simulink model "flocking"  (R2018b)
settings: Solver=FixedStepAuto  StartTime=0.0  StopTime=10  FixedStep=continuous_h  RelTol=1e-3
undefined symbols (not defined in the file or in its folder): continuous_h, traj
libraries: simulink x3, cf_lib x1, flocking_lib x1, vel_controller_lib x1
settings Model: Creator=sebbe  LastModifiedBy=sebbe

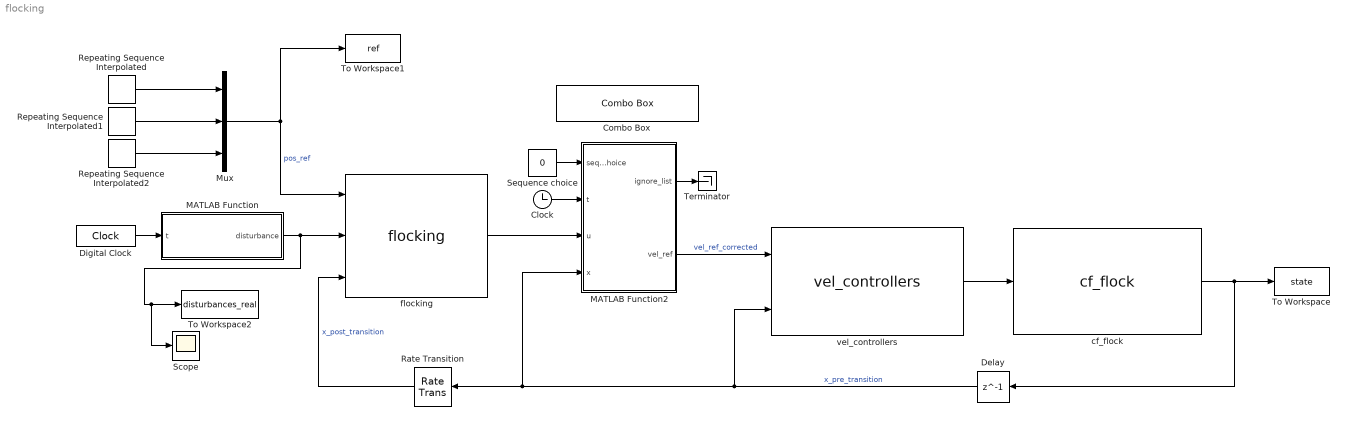
== system flocking ==
  Clock : Clock
  Combo Box : ComboBox  WebBlockId=48  SelectedLabel=Disabled
      settings: Values={{'Disabled', 'Merge 2', 'Fly Through', 'Hover'}, [0 1 2 3]}
  Delay : Delay  DelayLength=1
  Digital Clock : DigitalClock  SampleTime=continuous_h
  MATLAB Function : MATLAB Function  TreatAsAtomicUnit=on
  MATLAB Function2 : MATLAB Function  TreatAsAtomicUnit=on
  Mux : Mux  Inputs=3
  Rate Transition : RateTransition  OutPortSampleTime=0.05
  Repeating Sequence Interpolated : simulink/Sources/Repeating Sequence Interpolated  OutValues=traj.seq(1,:)'  TimeValues=traj.seq_t'  LookUpMeth=Interpolation-Use End Values  tsamp=continuous_h  OutMin=[]  OutMax=[]  OutDataTypeStr=double  OutputDataTypeScalingMode=double  OutDataType=fixdt(0,8)  OutScaling=2^-10
  Repeating Sequence Interpolated1 : simulink/Sources/Repeating Sequence Interpolated  OutValues=traj.seq(2,:)'  TimeValues=traj.seq_t'  LookUpMeth=Interpolation-Use End Values  tsamp=continuous_h  OutMin=[]  OutMax=[]  OutDataTypeStr=double  OutputDataTypeScalingMode=double  OutDataType=fixdt(0,8)  OutScaling=2^-10
  Repeating Sequence Interpolated2 : simulink/Sources/Repeating Sequence Interpolated  OutValues=traj.seq(3,:)'  TimeValues=traj.seq_t'  LookUpMeth=Interpolation-Use End Values  tsamp=continuous_h  OutMin=[]  OutMax=[]  OutDataTypeStr=double  OutputDataTypeScalingMode=double  OutDataType=fixdt(0,8)  OutScaling=2^-10
  Scope : Scope
  Sequence choice : Constant  Value=0
  Terminator : Terminator
  To Workspace : ToWorkspace  VariableName=state  SaveFormat=Timeseries  SampleTime=continuous_h
  To Workspace1 : ToWorkspace  VariableName=ref  SaveFormat=Timeseries  SampleTime=continuous_h
  To Workspace2 : ToWorkspace  VariableName=disturbances_real  SaveFormat=Timeseries  SampleTime=-1
  cf_flock : cf_lib/cf_flock  SystemSampleTime=-1
  flocking : flocking_lib/flocking  SystemSampleTime=-1
  vel_controllers : vel_controller_lib/vel_controllers  SystemSampleTime=-1
  wires:
  vel_controllers/1 -> cf_flock/1
  cf_flock/1 -> Delay/1, To Workspace/1
  Delay/1 -> vel_controllers/2, MATLAB Function2/4(x), Rate Transition/1  "x_pre_transition"
  Repeating Sequence Interpolated1/1 -> Mux/2
  Mux/1 -> flocking/1, To Workspace1/1  "pos_ref"
  Repeating Sequence Interpolated2/1 -> Mux/3
  Repeating Sequence Interpolated/1 -> Mux/1
  Digital Clock/1 -> MATLAB Function/1(t)
  MATLAB Function/1(disturbance) -> flocking/2, Scope/1, To Workspace2/1
  Clock/1 -> MATLAB Function2/2(t)
  MATLAB Function2/2(vel_ref) -> vel_controllers/1  "vel_ref_corrected"
  Sequence choice/1 -> MATLAB Function2/1(sequence_choice)
  Rate Transition/1 -> flocking/3  "x_post_transition"
  flocking/1 -> MATLAB Function2/3(u)
  MATLAB Function2/1(ignore_list) -> Terminator/1

== matlab function flocking/MATLAB Function ==
  data: t input; disturbances parameter; disturbance output
function disturbance = dynamic_disturbance(t, disturbances)
disturbance = disturbances;
%disturbance(3,1) = disturbances(3,1) - 49.6 + 30*t - 9.82*t^2/2;
%disturbance(1,1) = disturbances(1,1) - 3 + 1*t;

== matlab function flocking/MATLAB Function2 ==
  data: ignore_list output; sequence_choice input; t input; u input; vel_ref output; x input
function [ignore_list, vel_ref] = intercept_ref(sequence_choice, t, u, x)
vel_ref = u;
ignore_list = [0];
if sequence_choice == 0
    return
end

[n_states, N] = size(x);

switch sequence_choice
    case 1 % Merge 2
        if t < 6
            r = [0; -1; 1];
            e = r - x(1:3,1);
            vel_ref(:,1) = 0.5*e;
        end
        
    case 2 % Fly through
        r = [2; 0; 1];
        e = r - x(1:3,1);
        vel_ref(:,1) = 0.5*e;
    case 3 % Hover
        pos_hover = [0 0 0.96;
            0.52 0 1.02;
            0 0.48 0.98;
            -0.55 0 1;
            0 -0.51 1];
        if t < 6
            for n=1:N
                r = pos_hover(n,:)';
                e = r - x(1:3,n);
                vel_ref(:,n) = 0.5*e;
            end
        end
    otherwise
        return

end
